simulink model "PMDC_H11"  (R2025a)
settings: Solver=VariableStepAuto  StartTime=0.0  StopTime=50e-3  MaxStep=329e-6/25  RelTol=1e-3
settings Model: Creator=Szalay  LastModifiedBy=Szalay

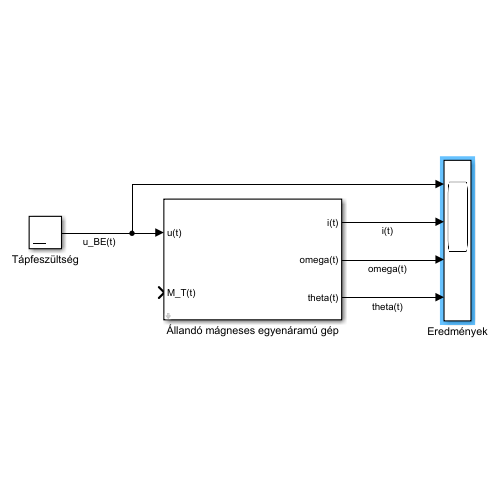
[thumbnail: Simulink's stored preview of the top-level diagram]
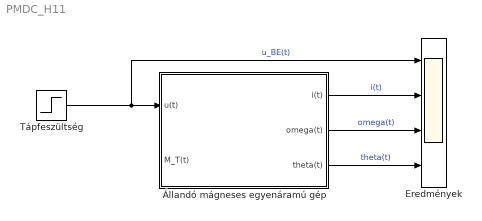
== system PMDC_H11 ==
  Eredmények : Scope  NumInputPorts=4
      settings: ActiveDisplayYMinimum=-1.4999999999999996  ActiveDisplayYMaximum=13.5
  Tápfeszültség : Step  Time=1e-3  After=12  SampleTime=0
  Állandó mágneses egyenáramú gép : Subsystem  mask(Állandó mágneses egyenáramú gép){R=79e-3, L=26e-6, k_E=13.7e-3, k_T=13.7e-3, J=99.5e-7, B=5.15e-6, i_0=0, omega_0=0, theta_0=0}
      mask prompts: R "Armatúra ellenállás"; L "Armatúra induktivitás"; k_E "Feszültségállandó"; k_T "Nyomatékállandó"; J "A forgórész tehetetlenségi nyomatéka"; B "Forgási súrlódási együttható"; i_0 "Kezdeti áramerősség"; omega_0 "Kezdeti szögsebesség"; theta_0 "Kezdeti szöghelyzet"
      mask help: Az állandó mágneses egyenáramú gép modellje a Maxon DCX 35L típus alapján paraméterezve.
      mask DialogControl Container4 Prompt: Modellparaméterek
      mask DialogControl Container6 Prompt: Villamos áramköri jellemzők
      mask DialogControl Container7 Prompt: Mágnesköri gépállandók
      mask DialogControl Container8 Prompt: A forgó részrendszer jellemzői
      mask DialogControl Container5 Prompt: Kezdeti értékek
      mask DialogControl Container9 Prompt: Villamos áramkör
      mask DialogControl Container10 Prompt: Forgó részrendszer
  wires:
  Tápfeszültség/1 -> Eredmények/1, Állandó mágneses egyenáramú gép/1(u(t))  "u_BE(t)"
  Állandó mágneses egyenáramú gép/1(i(t)) -> Eredmények/2  "i(t)"
  Állandó mágneses egyenáramú gép/2(omega(t)) -> Eredmények/3  "omega(t)"
  Állandó mágneses egyenáramú gép/3(theta(t)) -> Eredmények/4  "theta(t)"

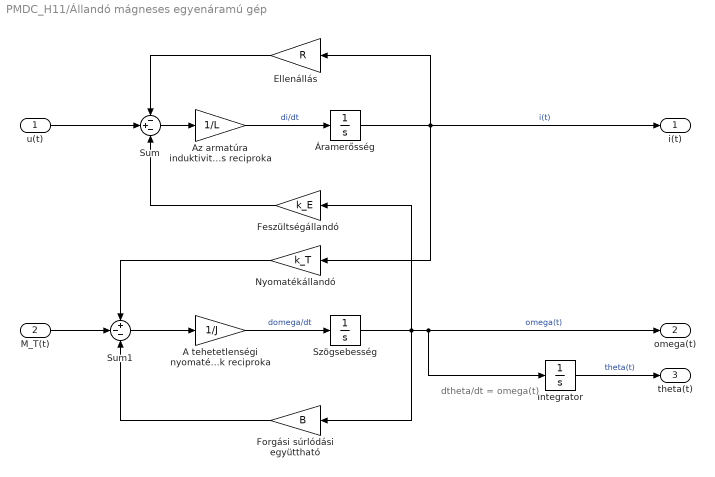
== system PMDC_H11/Állandó mágneses egyenáramú gép ==
  note: dtheta/dt = omega(t)
  u(t) : Inport
  M_T(t) : Inport  Port=2
  A tehetetlenségi nyomaték reciproka : Gain  Gain=1/J
  Az armatúra induktivitás reciproka : Gain  Gain=1/L
  Ellenállás : Gain  Gain=R
  Feszültségállandó : Gain  Gain=k_E
  Forgási súrlódási együttható : Gain  Gain=B
  Integrator : Integrator
  Nyomatékállandó : Gain  Gain=k_T
  Sum : Sum  Inputs=-+-
  Sum1 : Sum  Inputs=+--
  Szögsebesség : Integrator
  Áramerősség : Integrator
  i(t) : Outport
  omega(t) : Outport  Port=2
  theta(t) : Outport  Port=3
  wires:
  Szögsebesség/1 -> omega(t)/1, Integrator/1, Forgási súrlódási együttható/1, Feszültségállandó/1  "omega(t)"
  Forgási súrlódási együttható/1 -> Sum1/3
  Az armatúra induktivitás reciproka/1 -> Áramerősség/1  "di/dt"
  Sum1/1 -> A tehetetlenségi nyomaték reciproka/1
  Feszültségállandó/1 -> Sum/3
  Sum/1 -> Az armatúra induktivitás reciproka/1
  Ellenállás/1 -> Sum/1
  Áramerősség/1 -> i(t)/1, Ellenállás/1, Nyomatékállandó/1  "i(t)"
  Nyomatékállandó/1 -> Sum1/1
  u(t)/1 -> Sum/2
  A tehetetlenségi nyomaték reciproka/1 -> Szögsebesség/1  "domega/dt"
  M_T(t)/1 -> Sum1/2
  Integrator/1 -> theta(t)/1  "theta(t)"
